simulink model "model"  (R2014a)
(part 5 of 5)

      | %<Vbase>V
      | %<VLF>pu
      | %<angleLF>deg.
      | %<Name>
  bus38 : powerlib/Measurements/Load Flow Bus  LConnTagsString=a  ID=bus38  Vbase=230000  Vref=1  Vangle=0  VLF=1  angleLF=0
      settings: AttributesFormatString=|
      | %<ID>
      | %<Vbase>V
      | %<VLF>pu
      | %<angleLF>deg.
      | %<Name>
  bus39 : powerlib/Measurements/Load Flow Bus  LConnTagsString=a  ID=bus39  Vbase=230000  Vref=1  Vangle=0  VLF=1  angleLF=0
      settings: AttributesFormatString=|
      | %<ID>
      | %<Vbase>V
      | %<VLF>pu
      | %<angleLF>deg.
      | %<Name>
  bus4 : powerlib/Measurements/Load Flow Bus  LConnTagsString=a  ID=bus4  Vbase=66000  Vref=1  Vangle=0  VLF=1  angleLF=0
      settings: AttributesFormatString=|
      | %<ID>
      | %<Vbase>V
      | %<VLF>pu
      | %<angleLF>deg.
      | %<Name>
  bus40 : powerlib/Measurements/Load Flow Bus  LConnTagsString=a  ID=bus40  Vbase=230000  Vref=1  Vangle=0  VLF=1  angleLF=0
      settings: AttributesFormatString=|
      | %<ID>
      | %<Vbase>V
      | %<VLF>pu
      | %<angleLF>deg.
      | %<Name>
  bus41 : powerlib/Measurements/Load Flow Bus  LConnTagsString=a  ID=bus41  Vbase=230000  Vref=1  Vangle=0  VLF=1  angleLF=0
      settings: AttributesFormatString=|
      | %<ID>
      | %<Vbase>V
      | %<VLF>pu
      | %<angleLF>deg.
      | %<Name>
  bus42 : powerlib/Measurements/Load Flow Bus  LConnTagsString=a  ID=bus42  Vbase=230000  Vref=1  Vangle=0  VLF=1  angleLF=0
      settings: AttributesFormatString=|
      | %<ID>
      | %<Vbase>V
      | %<VLF>pu
      | %<angleLF>deg.
      | %<Name>
  bus43 : powerlib/Measurements/Load Flow Bus  LConnTagsString=a  ID=bus43  Vbase=230000  Vref=1  Vangle=0  VLF=1  angleLF=0
      settings: AttributesFormatString=|
      | %<ID>
      | %<Vbase>V
      | %<VLF>pu
      | %<angleLF>deg.
      | %<Name>
  bus44 : powerlib/Measurements/Load Flow Bus  LConnTagsString=a  ID=bus44  Vbase=230000  Vref=1  Vangle=0  VLF=1  angleLF=0
      settings: AttributesFormatString=|
      | %<ID>
      | %<Vbase>V
      | %<VLF>pu
      | %<angleLF>deg.
      | %<Name>
  bus45 : powerlib/Measurements/Load Flow Bus  LConnTagsString=a  ID=bus45  Vbase=230000  Vref=1  Vangle=0  VLF=1  angleLF=0
      settings: AttributesFormatString=|
      | %<ID>
      | %<Vbase>V
      | %<VLF>pu
      | %<angleLF>deg.
      | %<Name>
  bus46 : powerlib/Measurements/Load Flow Bus  LConnTagsString=a  ID=bus46  Vbase=230000  Vref=1  Vangle=0  VLF=1  angleLF=0
      settings: AttributesFormatString=|
      | %<ID>
      | %<Vbase>V
      | %<VLF>pu
      | %<angleLF>deg.
      | %<Name>
  bus47 : powerlib/Measurements/Load Flow Bus  LConnTagsString=a  ID=bus47  Vbase=230000  Vref=1  Vangle=0  VLF=1  angleLF=0
      settings: AttributesFormatString=|
      | %<ID>
      | %<Vbase>V
      | %<VLF>pu
      | %<angleLF>deg.
      | %<Name>
  bus48 : powerlib/Measurements/Load Flow Bus  LConnTagsString=a  ID=bus48  Vbase=230000  Vref=1  Vangle=0  VLF=1  angleLF=0
      settings: AttributesFormatString=|
      | %<ID>
      | %<Vbase>V
      | %<VLF>pu
      | %<angleLF>deg.
      | %<Name>
  bus49 : powerlib/Measurements/Load Flow Bus  LConnTagsString=a  ID=bus49  Vbase=230000  Vref=1  Vangle=0  VLF=1  angleLF=0
      settings: AttributesFormatString=|
      | %<ID>
      | %<Vbase>V
      | %<VLF>pu
      | %<angleLF>deg.
      | %<Name>
  bus5 : powerlib/Measurements/Load Flow Bus  LConnTagsString=a  ID=bus5  Vbase=66000  Vref=1  Vangle=0  VLF=1  angleLF=0
      settings: AttributesFormatString=|
      | %<ID>
      | %<Vbase>V
      | %<VLF>pu
      | %<angleLF>deg.
      | %<Name>
  bus50 : powerlib/Measurements/Load Flow Bus  LConnTagsString=a  ID=bus50  Vbase=230000  Vref=1  Vangle=0  VLF=1  angleLF=0
      settings: AttributesFormatString=|
      | %<ID>
      | %<Vbase>V
      | %<VLF>pu
      | %<angleLF>deg.
      | %<Name>
  bus51 : powerlib/Measurements/Load Flow Bus  LConnTagsString=a  ID=bus51  Vbase=230000  Vref=1  Vangle=0  VLF=1  angleLF=0
      settings: AttributesFormatString=|
      | %<ID>
      | %<Vbase>V
      | %<VLF>pu
      | %<angleLF>deg.
      | %<Name>
  bus52 : powerlib/Measurements/Load Flow Bus  LConnTagsString=a  ID=bus52  Vbase=230000  Vref=1  Vangle=0  VLF=1  angleLF=0
      settings: AttributesFormatString=|
      | %<ID>
      | %<Vbase>V
      | %<VLF>pu
      | %<angleLF>deg.
      | %<Name>
  bus53 : powerlib/Measurements/Load Flow Bus  LConnTagsString=a  ID=bus53  Vbase=230000  Vref=1  Vangle=0  VLF=1  angleLF=0
      settings: AttributesFormatString=|
      | %<ID>
      | %<Vbase>V
      | %<VLF>pu
      | %<angleLF>deg.
      | %<Name>
  bus54 : powerlib/Measurements/Load Flow Bus  LConnTagsString=a  ID=bus54  Vbase=230000  Vref=1  Vangle=0  VLF=1  angleLF=0
      settings: AttributesFormatString=|
      | %<ID>
      | %<Vbase>V
      | %<VLF>pu
      | %<angleLF>deg.
      | %<Name>
  bus55 : powerlib/Measurements/Load Flow Bus  LConnTagsString=a  ID=bus55  Vbase=230000  Vref=1  Vangle=0  VLF=1  angleLF=0
      settings: AttributesFormatString=|
      | %<ID>
      | %<Vbase>V
      | %<VLF>pu
      | %<angleLF>deg.
      | %<Name>
  bus56 : powerlib/Measurements/Load Flow Bus  LConnTagsString=a  ID=bus56  Vbase=230000  Vref=1  Vangle=0  VLF=1  angleLF=0
      settings: AttributesFormatString=|
      | %<ID>
      | %<Vbase>V
      | %<VLF>pu
      | %<angleLF>deg.
      | %<Name>
  bus57 : powerlib/Measurements/Load Flow Bus  LConnTagsString=a  ID=bus57  Vbase=230000  Vref=1  Vangle=0  VLF=1  angleLF=0
      settings: AttributesFormatString=|
      | %<ID>
      | %<Vbase>V
      | %<VLF>pu
      | %<angleLF>deg.
      | %<Name>
  bus58 : powerlib/Measurements/Load Flow Bus  LConnTagsString=a  ID=bus58  Vbase=230000  Vref=1  Vangle=0  VLF=1  angleLF=0
      settings: AttributesFormatString=|
      | %<ID>
      | %<Vbase>V
      | %<VLF>pu
      | %<angleLF>deg.
      | %<Name>
  bus59 : powerlib/Measurements/Load Flow Bus  LConnTagsString=a  ID=bus59  Vbase=230000  Vref=1  Vangle=0  VLF=1  angleLF=0
      settings: AttributesFormatString=|
      | %<ID>
      | %<Vbase>V
      | %<VLF>pu
      | %<angleLF>deg.
      | %<Name>
  bus6 : powerlib/Measurements/Load Flow Bus  LConnTagsString=a  ID=bus6  Vbase=66000  Vref=1  Vangle=0  VLF=1  angleLF=0
      settings: AttributesFormatString=|
      | %<ID>
      | %<Vbase>V
      | %<VLF>pu
      | %<angleLF>deg.
      | %<Name>
  bus60 : powerlib/Measurements/Load Flow Bus  LConnTagsString=a  ID=bus60  Vbase=230000  Vref=1  Vangle=0  VLF=1  angleLF=0
      settings: AttributesFormatString=|
      | %<ID>
      | %<Vbase>V
      | %<VLF>pu
      | %<angleLF>deg.
      | %<Name>
  bus61 : powerlib/Measurements/Load Flow Bus  LConnTagsString=a  ID=bus61  Vbase=230000  Vref=1  Vangle=0  VLF=1  angleLF=0
      settings: AttributesFormatString=|
      | %<ID>
      | %<Vbase>V
      | %<VLF>pu
      | %<angleLF>deg.
      | %<Name>
  bus62 : powerlib/Measurements/Load Flow Bus  LConnTagsString=a  ID=bus62  Vbase=230000  Vref=1  Vangle=0  VLF=1  angleLF=0
      settings: AttributesFormatString=|
      | %<ID>
      | %<Vbase>V
      | %<VLF>pu
      | %<angleLF>deg.
      | %<Name>
  bus63 : powerlib/Measurements/Load Flow Bus  LConnTagsString=a  ID=bus63  Vbase=230000  Vref=1  Vangle=0  VLF=1  angleLF=0
      settings: AttributesFormatString=|
      | %<ID>
      | %<Vbase>V
      | %<VLF>pu
      | %<angleLF>deg.
      | %<Name>
  bus64 : powerlib/Measurements/Load Flow Bus  LConnTagsString=a  ID=bus64  Vbase=230000  Vref=1  Vangle=0  VLF=1  angleLF=0
      settings: AttributesFormatString=|
      | %<ID>
      | %<Vbase>V
      | %<VLF>pu
      | %<angleLF>deg.
      | %<Name>
  bus65 : powerlib/Measurements/Load Flow Bus  LConnTagsString=a  ID=bus65  Vbase=230000  Vref=1  Vangle=0  VLF=1  angleLF=0
      settings: AttributesFormatString=|
      | %<ID>
      | %<Vbase>V
      | %<VLF>pu
      | %<angleLF>deg.
      | %<Name>
  bus66 : powerlib/Measurements/Load Flow Bus  LConnTagsString=a  ID=bus66  Vbase=230000  Vref=1  Vangle=0  VLF=1  angleLF=0
      settings: AttributesFormatString=|
      | %<ID>
      | %<Vbase>V
      | %<VLF>pu
      | %<angleLF>deg.
      | %<Name>
  bus67 : powerlib/Measurements/Load Flow Bus  LConnTagsString=a  ID=bus67  Vbase=230000  Vref=1  Vangle=0  VLF=1  angleLF=0
      settings: AttributesFormatString=|
      | %<ID>
      | %<Vbase>V
      | %<VLF>pu
      | %<angleLF>deg.
      | %<Name>
  bus68 : powerlib/Measurements/Load Flow Bus  LConnTagsString=a  ID=bus68  Vbase=230000  Vref=1  Vangle=0  VLF=1  angleLF=0
      settings: AttributesFormatString=|
      | %<ID>
      | %<Vbase>V
      | %<VLF>pu
      | %<angleLF>deg.
      | %<Name>
  bus69 : powerlib/Measurements/Load Flow Bus  LConnTagsString=a  ID=bus69  Vbase=230000  Vref=1  Vangle=0  VLF=1  angleLF=0
      settings: AttributesFormatString=|
      | %<ID>
      | %<Vbase>V
      | %<VLF>pu
      | %<angleLF>deg.
      | %<Name>
  bus7 : powerlib/Measurements/Load Flow Bus  LConnTagsString=a  ID=bus7  Vbase=66000  Vref=1  Vangle=0  VLF=1  angleLF=0
      settings: AttributesFormatString=|
      | %<ID>
      | %<Vbase>V
      | %<VLF>pu
      | %<angleLF>deg.
      | %<Name>
  bus70 : powerlib/Measurements/Load Flow Bus  LConnTagsString=a  ID=bus70  Vbase=230000  Vref=1  Vangle=0  VLF=1  angleLF=0
      settings: AttributesFormatString=|
      | %<ID>
      | %<Vbase>V
      | %<VLF>pu
      | %<angleLF>deg.
      | %<Name>
  bus71 : powerlib/Measurements/Load Flow Bus  LConnTagsString=a  ID=bus71  Vbase=230000  Vref=1  Vangle=0  VLF=1  angleLF=0
      settings: AttributesFormatString=|
      | %<ID>
      | %<Vbase>V
      | %<VLF>pu
      | %<angleLF>deg.
      | %<Name>
  bus72 : powerlib/Measurements/Load Flow Bus  LConnTagsString=a  ID=bus72  Vbase=230000  Vref=1  Vangle=0  VLF=1  angleLF=0
      settings: AttributesFormatString=|
      | %<ID>
      | %<Vbase>V
      | %<VLF>pu
      | %<angleLF>deg.
      | %<Name>
  bus73 : powerlib/Measurements/Load Flow Bus  LConnTagsString=a  ID=bus73  Vbase=230000  Vref=1  Vangle=0  VLF=1  angleLF=0
      settings: AttributesFormatString=|
      | %<ID>
      | %<Vbase>V
      | %<VLF>pu
      | %<angleLF>deg.
      | %<Name>
  bus74 : powerlib/Measurements/Load Flow Bus  LConnTagsString=a  ID=bus74  Vbase=230000  Vref=1  Vangle=0  VLF=1  angleLF=0
      settings: AttributesFormatString=|
      | %<ID>
      | %<Vbase>V
      | %<VLF>pu
      | %<angleLF>deg.
      | %<Name>
  bus75 : powerlib/Measurements/Load Flow Bus  LConnTagsString=a  ID=bus75  Vbase=230000  Vref=1  Vangle=0  VLF=1  angleLF=0
      settings: AttributesFormatString=|
      | %<ID>
      | %<Vbase>V
      | %<VLF>pu
      | %<angleLF>deg.
      | %<Name>
  bus76 : powerlib/Measurements/Load Flow Bus  LConnTagsString=a  ID=bus76  Vbase=230000  Vref=1  Vangle=0  VLF=1  angleLF=0
      settings: AttributesFormatString=|
      | %<ID>
      | %<Vbase>V
      | %<VLF>pu
      | %<angleLF>deg.
      | %<Name>
  bus77 : powerlib/Measurements/Load Flow Bus  LConnTagsString=a  ID=bus77  Vbase=230000  Vref=1  Vangle=0  VLF=1  angleLF=0
      settings: AttributesFormatString=|
      | %<ID>
      | %<Vbase>V
      | %<VLF>pu
      | %<angleLF>deg.
      | %<Name>
  bus78 : powerlib/Measurements/Load Flow Bus  LConnTagsString=a  ID=bus78  Vbase=230000  Vref=1  Vangle=0  VLF=1  angleLF=0
      settings: AttributesFormatString=|
      | %<ID>
      | %<Vbase>V
      | %<VLF>pu
      | %<angleLF>deg.
      | %<Name>
  bus79 : powerlib/Measurements/Load Flow Bus  LConnTagsString=a  ID=bus79  Vbase=230000  Vref=1  Vangle=0  VLF=1  angleLF=0
      settings: AttributesFormatString=|
      | %<ID>
      | %<Vbase>V
      | %<VLF>pu
      | %<angleLF>deg.
      | %<Name>
  bus8 : powerlib/Measurements/Load Flow Bus  LConnTagsString=a  ID=bus8  Vbase=66000  Vref=1  Vangle=0  VLF=1  angleLF=0
      settings: AttributesFormatString=|
      | %<ID>
      | %<Vbase>V
      | %<VLF>pu
      | %<angleLF>deg.
      | %<Name>
  bus80 : powerlib/Measurements/Load Flow Bus  LConnTagsString=a  ID=bus80  Vbase=230000  Vref=1  Vangle=0  VLF=1  angleLF=0
      settings: AttributesFormatString=|
      | %<ID>
      | %<Vbase>V
      | %<VLF>pu
      | %<angleLF>deg.
      | %<Name>
  bus81 : powerlib/Measurements/Load Flow Bus  LConnTagsString=a  ID=bus81  Vbase=230000  Vref=1  Vangle=0  VLF=1  angleLF=0
      settings: AttributesFormatString=|
      | %<ID>
      | %<Vbase>V
      | %<VLF>pu
      | %<angleLF>deg.
      | %<Name>
  bus82 : powerlib/Measurements/Load Flow Bus  LConnTagsString=a  ID=bus82  Vbase=230000  Vref=1  Vangle=0  VLF=1  angleLF=0
      settings: AttributesFormatString=|
      | %<ID>
      | %<Vbase>V
      | %<VLF>pu
      | %<angleLF>deg.
      | %<Name>
  bus83 : powerlib/Measurements/Load Flow Bus  LConnTagsString=a  ID=bus83  Vbase=230000  Vref=1  Vangle=0  VLF=1  angleLF=0
      settings: AttributesFormatString=|
      | %<ID>
      | %<Vbase>V
      | %<VLF>pu
      | %<angleLF>deg.
      | %<Name>
  bus84 : powerlib/Measurements/Load Flow Bus  LConnTagsString=a  ID=bus84  Vbase=230000  Vref=1  Vangle=0  VLF=1  angleLF=0
      settings: AttributesFormatString=|
      | %<ID>
      | %<Vbase>V
      | %<VLF>pu
      | %<angleLF>deg.
      | %<Name>
  bus85 : powerlib/Measurements/Load Flow Bus  LConnTagsString=a  ID=bus85  Vbase=230000  Vref=1  Vangle=0  VLF=1  angleLF=0
      settings: AttributesFormatString=|
      | %<ID>
      | %<Vbase>V
      | %<VLF>pu
      | %<angleLF>deg.
      | %<Name>
  bus86 : powerlib/Measurements/Load Flow Bus  LConnTagsString=a  ID=bus86  Vbase=400000  Vref=1  Vangle=0  VLF=1  angleLF=0
      settings: AttributesFormatString=|
      | %<ID>
      | %<Vbase>V
      | %<VLF>pu
      | %<angleLF>deg.
      | %<Name>
  bus87 : powerlib/Measurements/Load Flow Bus  LConnTagsString=a  ID=bus87  Vbase=400000  Vref=1  Vangle=0  VLF=1  angleLF=0
      settings: AttributesFormatString=|
      | %<ID>
      | %<Vbase>V
      | %<VLF>pu
      | %<angleLF>deg.
      | %<Name>
  bus88 : powerlib/Measurements/Load Flow Bus  LConnTagsString=a  ID=bus88  Vbase=400000  Vref=1  Vangle=0  VLF=1  angleLF=0
      settings: AttributesFormatString=|
      | %<ID>
      | %<Vbase>V
      | %<VLF>pu
      | %<angleLF>deg.
      | %<Name>
  bus89 : powerlib/Measurements/Load Flow Bus  LConnTagsString=a  ID=bus89  Vbase=400000  Vref=1  Vangle=0  VLF=1  angleLF=0
      settings: AttributesFormatString=|
      | %<ID>
      | %<Vbase>V
      | %<VLF>pu
      | %<angleLF>deg.
      | %<Name>
  bus9 : powerlib/Measurements/Load Flow Bus  LConnTagsString=a  ID=bus9  Vbase=66000  Vref=1  Vangle=0  VLF=1  angleLF=0
      settings: AttributesFormatString=|
      | %<ID>
      | %<Vbase>V
      | %<VLF>pu
      | %<angleLF>deg.
      | %<Name>
  bus90 : powerlib/Measurements/Load Flow Bus  LConnTagsString=a  ID=bus90  Vbase=400000  Vref=1  Vangle=0  VLF=1  angleLF=0
      settings: AttributesFormatString=|
      | %<ID>
      | %<Vbase>V
      | %<VLF>pu
      | %<angleLF>deg.
      | %<Name>
  bus91 : powerlib/Measurements/Load Flow Bus  LConnTagsString=a  ID=bus91  Vbase=400000  Vref=1  Vangle=0  VLF=1  angleLF=0
      settings: AttributesFormatString=|
      | %<ID>
      | %<Vbase>V
      | %<VLF>pu
      | %<angleLF>deg.
      | %<Name>
  bus92 : powerlib/Measurements/Load Flow Bus  LConnTagsString=a  ID=bus92  Vbase=400000  Vref=1  Vangle=0  VLF=1  angleLF=0
      settings: AttributesFormatString=|
      | %<ID>
      | %<Vbase>V
      | %<VLF>pu
      | %<angleLF>deg.
      | %<Name>
  bus93 : powerlib/Measurements/Load Flow Bus  LConnTagsString=a  ID=bus93  Vbase=400000  Vref=1  Vangle=0  VLF=1  angleLF=0
      settings: AttributesFormatString=|
      | %<ID>
      | %<Vbase>V
      | %<VLF>pu
      | %<angleLF>deg.
      | %<Name>
  bus94 : powerlib/Measurements/Load Flow Bus  LConnTagsString=a  ID=bus94  Vbase=400000  Vref=1  Vangle=0  VLF=1  angleLF=0
      settings: AttributesFormatString=|
      | %<ID>
      | %<Vbase>V
      | %<VLF>pu
      | %<angleLF>deg.
      | %<Name>
  bus95 : powerlib/Measurements/Load Flow Bus  LConnTagsString=a  ID=bus95  Vbase=400000  Vref=1  Vangle=0  VLF=1  angleLF=0
      settings: AttributesFormatString=|
      | %<ID>
      | %<Vbase>V
      | %<VLF>pu
      | %<angleLF>deg.
      | %<Name>
  bus96 : powerlib/Measurements/Load Flow Bus  LConnTagsString=a  ID=bus96  Vbase=400000  Vref=1  Vangle=0  VLF=1  angleLF=0
      settings: AttributesFormatString=|
      | %<ID>
      | %<Vbase>V
      | %<VLF>pu
      | %<angleLF>deg.
      | %<Name>
  bus97 : powerlib/Measurements/Load Flow Bus  LConnTagsString=a  ID=bus97  Vbase=400000  Vref=1  Vangle=0  VLF=1  angleLF=0
      settings: AttributesFormatString=|
      | %<ID>
      | %<Vbase>V
      | %<VLF>pu
      | %<angleLF>deg.
      | %<Name>
  bus98 : powerlib/Measurements/Load Flow Bus  LConnTagsString=a  ID=bus98  Vbase=400000  Vref=1  Vangle=0  VLF=1  angleLF=0
      settings: AttributesFormatString=|
      | %<ID>
      | %<Vbase>V
      | %<VLF>pu
      | %<angleLF>deg.
      | %<Name>
  bus99 : powerlib/Measurements/Load Flow Bus  LConnTagsString=a  ID=bus99  Vbase=66000  Vref=1  Vangle=0  VLF=1  angleLF=0
      settings: AttributesFormatString=|
      | %<ID>
      | %<Vbase>V
      | %<VLF>pu
      | %<angleLF>deg.
      | %<Name>
  powergui : powerlib/powergui  Priority=1  SimulationMode=Continuous  SolverType=Tustin  SampleTime=50e-6  frequency=60  SPID=off  DisableSnubberDevices=off  DisableRonSwitches=off  DisableVfSwitches=off  SwTol=0  Interpol=off  DisplayEquations=off  Ts=0  methode=off  frequencyindice=60  Pbase=100e6  ErrMax=1e-4  Iterations=50  UnitsV=kV  UnitsW=MW  FunctionMessages=off  echomessages=off  HookPort=off  EnableUseOfTLC=off  x0status=blocks  RestoreLinks=warning  ResistiveCurrentMeasurement=off  Frange=[0:2:500]  Ylog=off  Xlog=on  ShowGrid=off  save=off  variable=ZData  structure=0  ZoomFFT=off  StartTime=0.0  cycles=1  DisplayStyle=1  fundamental=60  FreqAxis=off  MaxFrequency=1000  frequencyindicesteady=1  RmsSteady=1  display=off
  Ötztal___Zirl_CN_147563007_110000_CN_100404264_110000 : powerlib/Elements/Distributed Parameters Line  Phases=3  Frequency=60  Resistance=[0.01273 0.3864]  Inductance="[0.9337e-3  4.1264e-3]"  Capacitance=[12.74e-9 7.751e-9]  Length=100  x1=[0 0 0 0; 0.0001244 0 0 0; 0.0002488 0 0 0; 0.0003733 0 0 0; 0.0004977 0 0 0; 0.0006221 0 0 0]  x2=[0 0 0 0; 0.0001244 0 0 0; 0.0002488 0 0 0; 0.0003733 0 0 0; 0.0004977 0 0 0; 0.0006221 0 0 0]  x3=[0 0 0 0; 0.0001244 0 0 0; 0.0002488 0 0 0; 0.0003733 0 0 0; 0.0004977 0 0 0; 0.0006221 0 0 0]  x4=[0 0 0 0; 0.0001244 0 0 0; 0.0002488 0 0 0; 0.0003733 0 0 0; 0.0004977 0 0 0; 0.0006221 0 0 0]  x5=0  V1=ones(3,3)  V2=ones(3,3)  I1=ones(3,3)  I2=ones(3,3)  nHarmo=1  Measurements=None
  connections:
  T_172436615__/LConn1 -- _CN_172436615_66000_CN_150358740_66000/LConn1
  T_172436615__/LConn2 -- _CN_172436615_66000_CN_150358740_66000/LConn2
  _CN_172436615_66000_CN_150358740_66000/LConn3 -- T_172436615__/LConn3 -- bus1/LConn1
  _CN_172436615_66000_CN_150358740_66000/RConn1 -- T_150358740__/LConn1 -- _CN_153750231_66000_CN_150358740_66000/LConn1
  _CN_172436615_66000_CN_150358740_66000/RConn2 -- T_150358740__/LConn2 -- _CN_153750231_66000_CN_150358740_66000/LConn2
  _CN_172436615_66000_CN_150358740_66000/RConn3 -- T_150358740__/LConn3 -- _CN_153750231_66000_CN_150358740_66000/LConn3 -- bus2/LConn1
  _CN_152303368_66000_CN_152303372_66000/LConn1 -- T_152303368__/LConn1 -- _CN_152303368_66000_CN_152322299_66000/LConn1
  _CN_152303368_66000_CN_152303372_66000/LConn2 -- T_152303368__/LConn2 -- _CN_152303368_66000_CN_152322299_66000/LConn2
  _CN_152303368_66000_CN_152303372_66000/LConn3 -- T_152303368__/LConn3 -- _CN_152303368_66000_CN_152322299_66000/LConn3 -- bus3/LConn1
  _CN_152303368_66000_CN_152303372_66000/RConn1 -- T_152303372__/RConn1 -- _CN_152303372_66000_CN_154474061_66000/LConn1 -- _CN_152303372_66000_CN_150256289_66000/LConn1 -- L_152303372/LConn1
  _CN_152303368_66000_CN_152303372_66000/RConn2 -- T_152303372__/RConn2 -- _CN_152303372_66000_CN_154474061_66000/LConn2 -- _CN_152303372_66000_CN_150256289_66000/LConn2 -- L_152303372/LConn2
  _CN_152303368_66000_CN_152303372_66000/RConn3 -- T_152303372__/RConn3 -- _CN_152303372_66000_CN_154474061_66000/LConn3 -- _CN_152303372_66000_CN_150256289_66000/LConn3 -- L_152303372/LConn3 -- bus4/LConn1
  T_152322299__/LConn1 -- _CN_152303368_66000_CN_152322299_66000/RConn1
  T_152322299__/LConn2 -- _CN_152303368_66000_CN_152322299_66000/RConn2
  _CN_152303368_66000_CN_152322299_66000/RConn3 -- T_152322299__/LConn3 -- bus5/LConn1
  _CN_130804490_66000_CN_223610661_66000/LConn1 -- T_130804490__/RConn1 -- _CN_130804490_66000_CN_130790482_66000/LConn1 -- _CN_130804490_66000_CN_382319714_66000/LConn1 -- L_130804490/LConn1
  _CN_130804490_66000_CN_223610661_66000/LConn2 -- T_130804490__/RConn2 -- _CN_130804490_66000_CN_130790482_66000/LConn2 -- _CN_130804490_66000_CN_382319714_66000/LConn2 -- L_130804490/LConn2
  _CN_130804490_66000_CN_223610661_66000/LConn3 -- T_130804490__/RConn3 -- _CN_130804490_66000_CN_130790482_66000/LConn3 -- _CN_130804490_66000_CN_382319714_66000/LConn3 -- L_130804490/LConn3 -- bus6/LConn1
  _CN_130804490_66000_CN_223610661_66000/RConn1 -- T_223610661__/LConn1 -- _CN_130790482_66000_CN_223610661_66000/LConn1
  _CN_130804490_66000_CN_223610661_66000/RConn2 -- T_223610661__/LConn2 -- _CN_130790482_66000_CN_223610661_66000/LConn2
  _CN_130804490_66000_CN_223610661_66000/RConn3 -- T_223610661__/LConn3 -- _CN_130790482_66000_CN_223610661_66000/LConn3 -- bus7/LConn1
  _CN_130804490_66000_CN_130790482_66000/RConn1 -- T_130790482__/LConn1 -- _CN_382484415_66000_CN_130790482_66000/LConn1 -- _CN_130790482_66000_CN_223610661_66000/RConn1 -- _CN_130790482_66000_CN_130805766_66000/LConn1
  _CN_130804490_66000_CN_130790482_66000/RConn2 -- T_130790482__/LConn2 -- _CN_382484415_66000_CN_130790482_66000/LConn2 -- _CN_130790482_66000_CN_223610661_66000/RConn2 -- _CN_130790482_66000_CN_130805766_66000/LConn2
  _CN_130804490_66000_CN_130790482_66000/RConn3 -- T_130790482__/LConn3 -- _CN_382484415_66000_CN_130790482_66000/LConn3 -- _CN_130790482_66000_CN_223610661_66000/RConn3 -- _CN_130790482_66000_CN_130805766_66000/LConn3 -- bus8/LConn1
  T_382319714__/LConn1 -- _CN_130804490_66000_CN_382319714_66000/RConn1
  T_382319714__/LConn2 -- _CN_130804490_66000_CN_382319714_66000/RConn2
  _CN_130804490_66000_CN_382319714_66000/RConn3 -- T_382319714__/LConn3 -- bus9/LConn1
  _CN_130804491_66000_CN_382489138_66000/LConn1 -- T_130804491__/RConn1 -- L_130804491/LConn1
  _CN_130804491_66000_CN_382489138_66000/LConn2 -- T_130804491__/RConn2 -- L_130804491/LConn2
  _CN_130804491_66000_CN_382489138_66000/LConn3 -- T_130804491__/RConn3 -- L_130804491/LConn3 -- bus10/LConn1
  G_382489138_/RConn1 -- _CN_130804491_66000_CN_382489138_66000/RConn1
  G_382489138_/RConn2 -- _CN_130804491_66000_CN_382489138_66000/RConn2
  _CN_130804491_66000_CN_382489138_66000/RConn3 -- G_382489138_/RConn3 -- bus11/LConn1
  T_154474061__/LConn1 -- _CN_152303372_66000_CN_154474061_66000/RConn1
  T_154474061__/LConn2 -- _CN_152303372_66000_CN_154474061_66000/RConn2
  _CN_152303372_66000_CN_154474061_66000/RConn3 -- T_154474061__/LConn3 -- bus12/LConn1
  _CN_152303372_66000_CN_150256289_66000/RConn1 -- T_150256289__/RConn1 -- _CN_150256289_66000_CN_171978321_66000/LConn1 -- L_150256289/LConn1 -- _CN_153750231_66000_CN_150256289_66000/LConn1
  _CN_152303372_66000_CN_150256289_66000/RConn2 -- T_150256289__/RConn2 -- _CN_150256289_66000_CN_171978321_66000/LConn2 -- L_150256289/LConn2 -- _CN_153750231_66000_CN_150256289_66000/LConn2
  _CN_152303372_66000_CN_150256289_66000/RConn3 -- T_150256289__/RConn3 -- _CN_150256289_66000_CN_171978321_66000/LConn3 -- L_150256289/LConn3 -- bus13/LConn1 -- _CN_153750231_66000_CN_150256289_66000/LConn3
  _CN_153750231_66000_CN_150256289_66000/RConn1 -- T_153750231__/LConn1 -- _CN_153750231_66000_CN_150358740_66000/RConn1
  _CN_153750231_66000_CN_150256289_66000/RConn2 -- T_153750231__/LConn2 -- _CN_153750231_66000_CN_150358740_66000/RConn2
  _CN_153750231_66000_CN_150256289_66000/RConn3 -- T_153750231__/LConn3 -- _CN_153750231_66000_CN_150358740_66000/RConn3 -- bus14/LConn1
  T_204550424__/LConn1 -- _CN_204550424_66000_CN_130805766_66000/LConn1
  T_204550424__/LConn2 -- _CN_204550424_66000_CN_130805766_66000/LConn2
  _CN_204550424_66000_CN_130805766_66000/LConn3 -- T_204550424__/LConn3 -- bus15/LConn1
  _CN_204550424_66000_CN_130805766_66000/RConn1 -- G_130805766_/RConn1 -- _CN_130790482_66000_CN_130805766_66000/RConn1 -- _CN_130805767_230000_CN_130805766_66000/LConn1 -- _CN_130804490_230000_CN_130805766_66000/LConn1 -- _CN_130804491_230000_CN_130805766_66000/LConn1 -- _CN_223610662_66000_CN_130805766_66000/LConn1
  _CN_204550424_66000_CN_130805766_66000/RConn2 -- G_130805766_/RConn2 -- _CN_130790482_66000_CN_130805766_66000/RConn2 -- _CN_130805767_230000_CN_130805766_66000/LConn2 -- _CN_130804490_230000_CN_130805766_66000/LConn2 -- _CN_130804491_230000_CN_130805766_66000/LConn2 -- _CN_223610662_66000_CN_130805766_66000/LConn2
  _CN_204550424_66000_CN_130805766_66000/RConn3 -- G_130805766_/RConn3 -- _CN_130790482_66000_CN_130805766_66000/RConn3 -- _CN_130805767_230000_CN_130805766_66000/LConn3 -- _CN_130804490_230000_CN_130805766_66000/LConn3 -- _CN_130804491_230000_CN_130805766_66000/LConn3 -- bus16/LConn1 -- _CN_223610662_66000_CN_130805766_66000/LConn3
  _CN_180326303_66000_CN_180330721_66000/LConn1 -- T_180326303__/RConn1 -- _CN_180326303_66000_CN_368593331_66000/LConn1 -- L_180326303/LConn1
  _CN_180326303_66000_CN_180330721_66000/LConn2 -- T_180326303__/RConn2 -- _CN_180326303_66000_CN_368593331_66000/LConn2 -- L_180326303/LConn2
  _CN_180326303_66000_CN_180330721_66000/LConn3 -- T_180326303__/RConn3 -- _CN_180326303_66000_CN_368593331_66000/LConn3 -- L_180326303/LConn3 -- bus17/LConn1
  T_180330721__/LConn1 -- _CN_180326303_66000_CN_180330721_66000/RConn1
  T_180330721__/LConn2 -- _CN_180326303_66000_CN_180330721_66000/RConn2
  _CN_180326303_66000_CN_180330721_66000/RConn3 -- T_180330721__/LConn3 -- bus18/LConn1
  T_368593331__/LConn1 -- _CN_180326303_66000_CN_368593331_66000/RConn1
  T_368593331__/LConn2 -- _CN_180326303_66000_CN_368593331_66000/RConn2
  _CN_180326303_66000_CN_368593331_66000/RConn3 -- T_368593331__/LConn3 -- bus19/LConn1
  _CN_150256289_66000_CN_171978321_66000/RConn1 -- T_171978321__/LConn1 -- _CN_171978319_66000_CN_171978321_66000/LConn1
  _CN_150256289_66000_CN_171978321_66000/RConn2 -- T_171978321__/LConn2 -- _CN_171978319_66000_CN_171978321_66000/LConn2
  _CN_150256289_66000_CN_171978321_66000/RConn3 -- T_171978321__/LConn3 -- _CN_171978319_66000_CN_171978321_66000/LConn3 -- bus20/LConn1
  _CN_167991716_66000_CN_157393020_66000/LConn1 -- T_167991716_66000_/LConn1 -- _CN_167991716_66000_CN_157858216_66000/LConn1
  _CN_167991716_66000_CN_157393020_66000/LConn2 -- T_167991716_66000_/LConn2 -- _CN_167991716_66000_CN_157858216_66000/LConn2
  _CN_167991716_66000_CN_157393020_66000/LConn3 -- T_167991716_66000_/LConn3 -- _CN_167991716_66000_CN_157858216_66000/LConn3 -- bus21/LConn1
  T_157393020__/LConn1 -- _CN_167991716_66000_CN_157393020_66000/RConn1
  T_157393020__/LConn2 -- _CN_167991716_66000_CN_157393020_66000/RConn2
  _CN_167991716_66000_CN_157393020_66000/RConn3 -- T_157393020__/LConn3 -- bus22/LConn1
  _CN_167991716_66000_CN_157858216_66000/RConn1 -- T_157858216_230000;66000_/RConn1 -- L_157858216/LConn1
  _CN_167991716_66000_CN_157858216_66000/RConn2 -- T_157858216_230000;66000_/RConn2 -- L_157858216/LConn2
  _CN_167991716_66000_CN_157858216_66000/RConn3 -- T_157858216_230000;66000_/RConn3 -- L_157858216/LConn3 -- bus23/LConn1
  _CN_223610662_66000_CN_130805766_66000/RConn1 -- T_223610662__/LConn1 -- _CN_223610662_66000_CN_382300120_66000/LConn1
  _CN_223610662_66000_CN_130805766_66000/RConn2 -- T_223610662__/LConn2 -- _CN_223610662_66000_CN_382300120_66000/LConn2
  _CN_223610662_66000_CN_130805766_66000/RConn3 -- T_223610662__/LConn3 -- _CN_223610662_66000_CN_382300120_66000/LConn3 -- bus24/LConn1
  T_382300120__/LConn1 -- _CN_223610662_66000_CN_382300120_66000/RConn1
  T_382300120__/LConn2 -- _CN_223610662_66000_CN_382300120_66000/RConn2
  _CN_223610662_66000_CN_382300120_66000/RConn3 -- T_382300120__/LConn3 -- bus25/LConn1
  T_382331561__/LConn1 -- _CN_382331561_66000_CN_131421941_66000/LConn1
  T_382331561__/LConn2 -- _CN_382331561_66000_CN_131421941_66000/LConn2
  _CN_382331561_66000_CN_131421941_66000/LConn3 -- T_382331561__/LConn3 -- bus26/LConn1
  _CN_382331561_66000_CN_131421941_66000/RConn1 -- T_131421941__/RConn1 -- L_131421941/LConn1
  _CN_382331561_66000_CN_131421941_66000/RConn2 -- T_131421941__/RConn2 -- L_131421941/LConn2
  _CN_382331561_66000_CN_131421941_66000/RConn3 -- T_131421941__/RConn3 -- L_131421941/LConn3 -- bus27/LConn1
  _CN_238298034_66000_CN_382898922_66000/LConn1 -- T_238298034__/RConn1 -- L_238298034/LConn1
  _CN_238298034_66000_CN_382898922_66000/LConn2 -- T_238298034__/RConn2 -- L_238298034/LConn2
  _CN_238298034_66000_CN_382898922_66000/LConn3 -- T_238298034__/RConn3 -- L_238298034/LConn3 -- bus28/LConn1
  T_382898922__/LConn1 -- _CN_238298034_66000_CN_382898922_66000/RConn1
  T_382898922__/LConn2 -- _CN_238298034_66000_CN_382898922_66000/RConn2
  _CN_238298034_66000_CN_382898922_66000/RConn3 -- T_382898922__/LConn3 -- bus29/LConn1
  T_382484415__/LConn1 -- _CN_382484415_66000_CN_130790482_66000/RConn1
  T_382484415__/LConn2 -- _CN_382484415_66000_CN_130790482_66000/RConn2
  _CN_382484415_66000_CN_130790482_66000/RConn3 -- T_382484415__/LConn3 -- bus30/LConn1
  _CN_150974532_66000_CN_155496431_66000/LConn1 -- T_150974532__/RConn1 -- L_150974532/LConn1
  _CN_150974532_66000_CN_155496431_66000/LConn2 -- T_150974532__/RConn2 -- L_150974532/LConn2
  _CN_150974532_66000_CN_155496431_66000/LConn3 -- T_150974532__/RConn3 -- L_150974532/LConn3 -- bus31/LConn1
  T_155496431__/LConn1 -- _CN_150974532_66000_CN_155496431_66000/RConn1
  T_155496431__/LConn2 -- _CN_150974532_66000_CN_155496431_66000/RConn2
  _CN_150974532_66000_CN_155496431_66000/RConn3 -- T_155496431__/LConn3 -- bus32/LConn1
  T_171978319__/LConn1 -- _CN_171978319_66000_CN_171978321_66000/RConn1
  T_171978319__/LConn2 -- _CN_171978319_66000_CN_171978321_66000/RConn2
  _CN_171978319_66000_CN_171978321_66000/RConn3 -- T_171978319__/LConn3 -- bus33/LConn1
  _CN_133331795_66000_CN_160840191_66000/LConn1 -- T_133331795__/RConn1 -- L_133331795/LConn1
  _CN_133331795_66000_CN_160840191_66000/LConn2 -- T_133331795__/RConn2 -- L_133331795/LConn2
  _CN_133331795_66000_CN_160840191_66000/LConn3 -- T_133331795__/RConn3 -- L_133331795/LConn3 -- bus34/LConn1
  T_160840191__/LConn1 -- _CN_133331795_66000_CN_160840191_66000/RConn1
  T_160840191__/LConn2 -- _CN_133331795_66000_CN_160840191_66000/RConn2
  _CN_133331795_66000_CN_160840191_66000/RConn3 -- T_160840191__/LConn3 -- bus35/LConn1
  T_163711729__/LConn1 -- _CN_163711729_66000_CN_110461432_66000/LConn1
  T_163711729__/LConn2 -- _CN_163711729_66000_CN_110461432_66000/LConn2
  _CN_163711729_66000_CN_110461432_66000/LConn3 -- T_163711729__/LConn3 -- bus36/LConn1
  T_110461432__محطة_الكهرباء/LConn1 -- _CN_163711729_66000_CN_110461432_66000/RConn1
  T_110461432__محطة_الكهرباء/LConn2 -- _CN_163711729_66000_CN_110461432_66000/RConn2
  _CN_163711729_66000_CN_110461432_66000/RConn3 -- T_110461432__محطة_الكهرباء/LConn3 -- bus37/LConn1
  _CN_152322304_230000_CN_161969636_230000/LConn1 -- T_152322304__/RConn1 -- L_152322304/LConn1
  _CN_152322304_230000_CN_161969636_230000/LConn2 -- T_152322304__/RConn2 -- L_152322304/LConn2
  _CN_152322304_230000_CN_161969636_230000/LConn3 -- T_152322304__/RConn3 -- L_152322304/LConn3 -- bus38/LConn1
  T_161969636__/LConn1 -- _CN_152322304_230000_CN_161969636_230000/RConn1
  T_161969636__/LConn2 -- _CN_152322304_230000_CN_161969636_230000/RConn2
  _CN_152322304_230000_CN_161969636_230000/RConn3 -- T_161969636__/LConn3 -- bus39/LConn1
  T_164725547__/LConn1 -- _CN_164725547_230000_CN_195237417_230000/LConn1
  T_164725547__/LConn2 -- _CN_164725547_230000_CN_195237417_230000/LConn2
  _CN_164725547_230000_CN_195237417_230000/LConn3 -- T_164725547__/LConn3 -- bus40/LConn1
  T_195237417__/LConn1 -- _CN_164725547_230000_CN_195237417_230000/RConn1
  T_195237417__/LConn2 -- _CN_164725547_230000_CN_195237417_230000/RConn2
  _CN_164725547_230000_CN_195237417_230000/RConn3 -- T_195237417__/LConn3 -- bus41/LConn1
  _CN_130805767_230000_CN_130805766_66000/RConn1 -- T_130805767__/RConn1 -- L_130805767/LConn1
  _CN_130805767_230000_CN_130805766_66000/RConn2 -- T_130805767__/RConn2 -- L_130805767/LConn2
  _CN_130805767_230000_CN_130805766_66000/RConn3 -- T_130805767__/RConn3 -- L_130805767/LConn3 -- bus42/LConn1
  T_152303369__/LConn1 -- _CN_152303369_230000_CN_150638744_230000/LConn1
  T_152303369__/LConn2 -- _CN_152303369_230000_CN_150638744_230000/LConn2
  _CN_152303369_230000_CN_150638744_230000/LConn3 -- T_152303369__/LConn3 -- bus43/LConn1
  _CN_152303369_230000_CN_150638744_230000/RConn1 -- T_150638744__/RConn1 -- _CN_152303372_230000_CN_150638744_230000/LConn1 -- _CN_150638744_230000_CN_150256289_230000/LConn1 -- _CN_150638744_230000_CN_151913391_230000/LConn1 -- _CN_150638744_230000_CN_150358741_230000/LConn1 -- L_150638744/LConn1
  _CN_152303369_230000_CN_150638744_230000/RConn2 -- T_150638744__/RConn2 -- _CN_152303372_230000_CN_150638744_230000/LConn2 -- _CN_150638744_230000_CN_150256289_230000/LConn2 -- _CN_150638744_230000_CN_151913391_230000/LConn2 -- _CN_150638744_230000_CN_150358741_230000/LConn2 -- L_150638744/LConn2
  _CN_152303369_230000_CN_150638744_230000/RConn3 -- T_150638744__/RConn3 -- _CN_152303372_230000_CN_150638744_230000/LConn3 -- _CN_150638744_230000_CN_150256289_230000/LConn3 -- _CN_150638744_230000_CN_151913391_230000/LConn3 -- _CN_150638744_230000_CN_150358741_230000/LConn3 -- L_150638744/LConn3 -- bus44/LConn1
  _CN_130804490_230000_CN_130805766_66000/RConn1 -- T_130804490__/LConn1 -- _CN_130804490_230000_CN_131421941_230000/LConn1
  _CN_130804490_230000_CN_130805766_66000/RConn2 -- T_130804490__/LConn2 -- _CN_130804490_230000_CN_131421941_230000/LConn2
  _CN_130804490_230000_CN_130805766_66000/RConn3 -- T_130804490__/LConn3 -- _CN_130804490_230000_CN_131421941_230000/LConn3 -- bus45/LConn1
  T_131421941__/LConn1 -- _CN_130804490_230000_CN_131421941_230000/RConn1
  T_131421941__/LConn2 -- _CN_130804490_230000_CN_131421941_230000/RConn2
  _CN_130804490_230000_CN_131421941_230000/RConn3 -- T_131421941__/LConn3 -- bus46/LConn1
  _CN_130804491_230000_CN_180326303_230000/LConn1 -- T_130804491__/LConn1 -- _CN_130804491_230000_CN_130805766_66000/RConn1
  _CN_130804491_230000_CN_180326303_230000/LConn2 -- T_130804491__/LConn2 -- _CN_130804491_230000_CN_130805766_66000/RConn2
  _CN_130804491_230000_CN_180326303_230000/LConn3 -- T_130804491__/LConn3 -- _CN_130804491_230000_CN_130805766_66000/RConn3 -- bus47/LConn1
  _CN_130804491_230000_CN_180326303_230000/RConn1 -- T_180326303__/LConn1 -- _CN_180326303_230000_CN_330757612_230000/LConn1 -- _CN_180326303_230000_CN_180326309_230000/LConn1 -- _CN_180326303_230000_CN_113711692_230000/LConn1
  _CN_130804491_230000_CN_180326303_230000/RConn2 -- T_180326303__/LConn2 -- _CN_180326303_230000_CN_330757612_230000/LConn2 -- _CN_180326303_230000_CN_180326309_230000/LConn2 -- _CN_180326303_230000_CN_113711692_230000/LConn2
  _CN_130804491_230000_CN_180326303_230000/RConn3 -- T_180326303__/LConn3 -- _CN_180326303_230000_CN_330757612_230000/LConn3 -- _CN_180326303_230000_CN_180326309_230000/LConn3 -- _CN_180326303_230000_CN_113711692_230000/LConn3 -- bus48/LConn1
  T_152303372__/LConn1 -- _CN_152303372_230000_CN_150638744_230000/RConn1
  T_152303372__/LConn2 -- _CN_152303372_230000_CN_150638744_230000/RConn2
  _CN_152303372_230000_CN_150638744_230000/RConn3 -- T_152303372__/LConn3 -- bus49/LConn1
  _CN_254292628_230000_CN_133424212_230000/LConn1 -- T_254292628__/LConn1 -- _CN_254292628_230000_CN_254292629_230000/LConn1
  _CN_254292628_230000_CN_133424212_230000/LConn2 -- T_254292628__/LConn2 -- _CN_254292628_230000_CN_254292629_230000/LConn2
  _CN_254292628_230000_CN_133424212_230000/LConn3 -- T_254292628__/LConn3 -- _CN_254292628_230000_CN_254292629_230000/LConn3 -- bus50/LConn1
  _CN_254292628_230000_CN_133424212_230000/RConn1 -- T_133424212__/LConn1 -- _CN_133424203_230000_CN_133424212_230000/LConn1 -- _CN_133424212_230000_CN_168164591_230000/LConn1
  _CN_254292628_230000_CN_133424212_230000/RConn2 -- T_133424212__/LConn2 -- _CN_133424203_230000_CN_133424212_230000/LConn2 -- _CN_133424212_230000_CN_168164591_230000/LConn2
  _CN_254292628_230000_CN_133424212_230000/RConn3 -- T_133424212__/LConn3 -- _CN_133424203_230000_CN_133424212_230000/LConn3 -- _CN_133424212_230000_CN_168164591_230000/LConn3 -- bus51/LConn1
  T_254292629__/LConn1 -- _CN_254292628_230000_CN_254292629_230000/RConn1
  T_254292629__/LConn2 -- _CN_254292628_230000_CN_254292629_230000/RConn2
  _CN_254292628_230000_CN_254292629_230000/RConn3 -- T_254292629__/LConn3 -- bus52/LConn1
  _CN_150638744_230000_CN_150256289_230000/RConn1 -- T_150256289__/LConn1 -- _CN_150256289_230000_CN_130593618_230000/LConn1 -- _CN_150256289_230000_CN_150358741_230000/LConn1
  _CN_150638744_230000_CN_150256289_230000/RConn2 -- T_150256289__/LConn2 -- _CN_150256289_230000_CN_130593618_230000/LConn2 -- _CN_150256289_230000_CN_150358741_230000/LConn2
  _CN_150638744_230000_CN_150256289_230000/RConn3 -- T_150256289__/LConn3 -- _CN_150256289_230000_CN_130593618_230000/LConn3 -- _CN_150256289_230000_CN_150358741_230000/LConn3 -- bus53/LConn1
  _CN_150638744_230000_CN_151913391_230000/RConn1 -- T_151913391__/LConn1 -- _CN_151913391_230000_CN_160110669_230000/LConn1
  _CN_150638744_230000_CN_151913391_230000/RConn2 -- T_151913391__/LConn2 -- _CN_151913391_230000_CN_160110669_230000/LConn2
  _CN_150638744_230000_CN_151913391_230000/RConn3 -- T_151913391__/LConn3 -- _CN_151913391_230000_CN_160110669_230000/LConn3 -- bus54/LConn1
  _CN_150638744_230000_CN_150358741_230000/RConn1 -- T_150358741__/LConn1 -- _CN_150256289_230000_CN_150358741_230000/RConn1 -- _CN_150358741_230000_CN_154838308_230000/LConn1 -- _CN_150358741_230000_CN_150579316_230000/LConn1
  _CN_150638744_230000_CN_150358741_230000/RConn2 -- T_150358741__/LConn2 -- _CN_150256289_230000_CN_150358741_230000/RConn2 -- _CN_150358741_230000_CN_154838308_230000/LConn2 -- _CN_150358741_230000_CN_150579316_230000/LConn2
  _CN_150638744_230000_CN_150358741_230000/RConn3 -- T_150358741__/LConn3 -- _CN_150256289_230000_CN_150358741_230000/RConn3 -- _CN_150358741_230000_CN_154838308_230000/LConn3 -- _CN_150358741_230000_CN_150579316_230000/LConn3 -- bus55/LConn1
  _CN_180326303_230000_CN_330757612_230000/RConn1 -- T_330757612__/LConn1 -- _CN_238298034_230000_CN_330757612_230000/LConn1
  _CN_180326303_230000_CN_330757612_230000/RConn2 -- T_330757612__/LConn2 -- _CN_238298034_230000_CN_330757612_230000/LConn2
  _CN_180326303_230000_CN_330757612_230000/RConn3 -- T_330757612__/LConn3 -- _CN_238298034_230000_CN_330757612_230000/LConn3 -- bus56/LConn1
  T_180326309__Electrical_substation/LConn1 -- _CN_180326303_230000_CN_180326309_230000/RConn1
  T_180326309__Electrical_substation/LConn2 -- _CN_180326303_230000_CN_180326309_230000/RConn2
  _CN_180326303_230000_CN_180326309_230000/RConn3 -- T_180326309__Electrical_substation/LConn3 -- bus57/LConn1
  _CN_180326303_230000_CN_113711692_230000/RConn1 -- T_113711692__/LConn1 -- _CN_238298034_230000_CN_113711692_230000/LConn1
  _CN_180326303_230000_CN_113711692_230000/RConn2 -- T_113711692__/LConn2 -- _CN_238298034_230000_CN_113711692_230000/LConn2
  _CN_180326303_230000_CN_113711692_230000/RConn3 -- T_113711692__/LConn3 -- _CN_238298034_230000_CN_113711692_230000/LConn3 -- bus58/LConn1
  _CN_150256289_230000_CN_130593618_230000/RConn1 -- G_130593618_/RConn1 -- _CN_168164591_230000_CN_130593618_230000/LConn1 -- _CN_150974530_400000_CN_130593618_230000/LConn1 -- _CN_150638744_400000_CN_130593618_230000/LConn1 -- _CN_123913890_230000_CN_130593618_230000/LConn1 -- _CN_130592294_230000_CN_130593618_230000/LConn1 -- _CN_124803179_230000_CN_130593618_230000/LConn1
  _CN_150256289_230000_CN_130593618_230000/RConn2 -- G_130593618_/RConn2 -- _CN_168164591_230000_CN_130593618_230000/LConn2 -- _CN_150974530_400000_CN_130593618_230000/LConn2 -- _CN_150638744_400000_CN_130593618_230000/LConn2 -- _CN_123913890_230000_CN_130593618_230000/LConn2 -- _CN_130592294_230000_CN_130593618_230000/LConn2 -- _CN_124803179_230000_CN_130593618_230000/LConn2
  _CN_150256289_230000_CN_130593618_230000/RConn3 -- G_130593618_/RConn3 -- _CN_168164591_230000_CN_130593618_230000/LConn3 -- _CN_150974530_400000_CN_130593618_230000/LConn3 -- _CN_150638744_400000_CN_130593618_230000/LConn3 -- bus59/LConn1 -- _CN_123913890_230000_CN_130593618_230000/LConn3 -- _CN_130592294_230000_CN_130593618_230000/LConn3 -- _CN_124803179_230000_CN_130593618_230000/LConn3
  _CN_123913890_230000_CN_130592294_230000/LConn1 -- T_123913890__/LConn1 -- _CN_123913890_230000_CN_130593618_230000/RConn1
  _CN_123913890_230000_CN_130592294_230000/LConn2 -- T_123913890__/LConn2 -- _CN_123913890_230000_CN_130593618_230000/RConn2
  _CN_123913890_230000_CN_130592294_230000/LConn3 -- T_123913890__/LConn3 -- _CN_123913890_230000_CN_130593618_230000/RConn3 -- bus60/LConn1
  _CN_123913890_230000_CN_130592294_230000/RConn1 -- T_130592294__/LConn1 -- _CN_130592294_230000_CN_133331793_230000/LConn1 -- _CN_130592294_230000_CN_160279731_230000/LConn1 -- _CN_130592294_230000_CN_154838308_230000/LConn1 -- _CN_130592294_230000_CN_130593618_230000/RConn1
  _CN_123913890_230000_CN_130592294_230000/RConn2 -- T_130592294__/LConn2 -- _CN_130592294_230000_CN_133331793_230000/LConn2 -- _CN_130592294_230000_CN_160279731_230000/LConn2 -- _CN_130592294_230000_CN_154838308_230000/LConn2 -- _CN_130592294_230000_CN_130593618_230000/RConn2
  _CN_123913890_230000_CN_130592294_230000/RConn3 -- T_130592294__/LConn3 -- _CN_130592294_230000_CN_133331793_230000/LConn3 -- _CN_130592294_230000_CN_160279731_230000/LConn3 -- _CN_130592294_230000_CN_154838308_230000/LConn3 -- _CN_130592294_230000_CN_130593618_230000/RConn3 -- bus61/LConn1
  _CN_130592294_230000_CN_133331793_230000/RConn1 -- G_133331793_المحطة_الحرارية_Thermal_power_plant/RConn1 -- _CN_133432875_230000_CN_133331793_230000/LConn1 -- _CN_162588721_230000_CN_133331793_230000/LConn1 -- _CN_133331795_230000_CN_133331793_230000/LConn1
  _CN_130592294_230000_CN_133331793_230000/RConn2 -- G_133331793_المحطة_الحرارية_Thermal_power_plant/RConn2 -- _CN_133432875_230000_CN_133331793_230000/LConn2 -- _CN_162588721_230000_CN_133331793_230000/LConn2 -- _CN_133331795_230000_CN_133331793_230000/LConn2
  _CN_130592294_230000_CN_133331793_230000/RConn3 -- G_133331793_المحطة_الحرارية_Thermal_power_plant/RConn3 -- _CN_133432875_230000_CN_133331793_230000/LConn3 -- _CN_162588721_230000_CN_133331793_230000/LConn3 -- _CN_133331795_230000_CN_133331793_230000/LConn3 -- bus62/LConn1
  _CN_130592294_230000_CN_160279731_230000/RConn1 -- T_160279731__/RConn1 -- L_160279731/LConn1
  _CN_130592294_230000_CN_160279731_230000/RConn2 -- T_160279731__/RConn2 -- L_160279731/LConn2
  _CN_130592294_230000_CN_160279731_230000/RConn3 -- T_160279731__/RConn3 -- L_160279731/LConn3 -- bus63/LConn1
  _CN_130592294_230000_CN_154838308_230000/RConn1 -- G_154838308_Al_Zara_Thermal_Power_Plant/RConn1 -- _CN_150358741_230000_CN_154838308_230000/RConn1 -- _CN_124803179_230000_CN_154838308_230000/LConn1
  _CN_130592294_230000_CN_154838308_230000/RConn2 -- G_154838308_Al_Zara_Thermal_Power_Plant/RConn2 -- _CN_150358741_230000_CN_154838308_230000/RConn2 -- _CN_124803179_230000_CN_154838308_230000/LConn2
  _CN_130592294_230000_CN_154838308_230000/RConn3 -- G_154838308_Al_Zara_Thermal_Power_Plant/RConn3 -- _CN_150358741_230000_CN_154838308_230000/RConn3 -- _CN_124803179_230000_CN_154838308_230000/LConn3 -- bus64/LConn1
  _CN_157858216_230000_CN_117335600_230000/LConn1 -- T_157858216_230000;66000_/LConn1 -- _CN_157858216_230000_CN_164701658_230000/LConn1
  _CN_157858216_230000_CN_117335600_230000/LConn2 -- T_157858216_230000;66000_/LConn2 -- _CN_157858216_230000_CN_164701658_230000/LConn2
  _CN_157858216_230000_CN_117335600_230000/LConn3 -- T_157858216_230000;66000_/LConn3 -- _CN_157858216_230000_CN_164701658_230000/LConn3 -- bus65/LConn1
  _CN_157858216_230000_CN_117335600_230000/RConn1 -- T_117335600_400000;230000_/RConn1 -- L_117335600/LConn1
  _CN_157858216_230000_CN_117335600_230000/RConn2 -- T_117335600_400000;230000_/RConn2 -- L_117335600/LConn2
  _CN_157858216_230000_CN_117335600_230000/RConn3 -- T_117335600_400000;230000_/RConn3 -- L_117335600/LConn3 -- bus66/LConn1
  T_164701658__/LConn1 -- _CN_157858216_230000_CN_164701658_230000/RConn1
  T_164701658__/LConn2 -- _CN_157858216_230000_CN_164701658_230000/RConn2
  _CN_157858216_230000_CN_164701658_230000/RConn3 -- T_164701658__/LConn3 -- bus67/LConn1
  T_133432875__/LConn1 -- _CN_133432875_230000_CN_133331793_230000/RConn1
  T_133432875__/LConn2 -- _CN_133432875_230000_CN_133331793_230000/RConn2
  _CN_133432875_230000_CN_133331793_230000/RConn3 -- T_133432875__/LConn3 -- bus68/LConn1
  _CN_205359278_230000_CN_204311935_230000/LConn1 -- T_205359278__/LConn1 -- _CN_205359278_230000_CN_160110669_230000/LConn1
  _CN_205359278_230000_CN_204311935_230000/LConn2 -- T_205359278__/LConn2 -- _CN_205359278_230000_CN_160110669_230000/LConn2
  _CN_205359278_230000_CN_204311935_230000/LConn3 -- T_205359278__/LConn3 -- _CN_205359278_230000_CN_160110669_230000/LConn3 -- bus69/LConn1
  T_204311935__/LConn1 -- _CN_205359278_230000_CN_204311935_230000/RConn1
  T_204311935__/LConn2 -- _CN_205359278_230000_CN_204311935_230000/RConn2
  _CN_205359278_230000_CN_204311935_230000/RConn3 -- T_204311935__/LConn3 -- bus70/LConn1
  _CN_205359278_230000_CN_160110669_230000/RConn1 -- T_160110669__/LConn1 -- _CN_163811126_230000_CN_160110669_230000/LConn1 -- _CN_160110669_230000_CN_160110681_230000/LConn1 -- _CN_151913391_230000_CN_160110669_230000/RConn1
  _CN_205359278_230000_CN_160110669_230000/RConn2 -- T_160110669__/LConn2 -- _CN_163811126_230000_CN_160110669_230000/LConn2 -- _CN_160110669_230000_CN_160110681_230000/LConn2 -- _CN_151913391_230000_CN_160110669_230000/RConn2
  _CN_205359278_230000_CN_160110669_230000/RConn3 -- T_160110669__/LConn3 -- _CN_163811126_230000_CN_160110669_230000/LConn3 -- _CN_160110669_230000_CN_160110681_230000/LConn3 -- bus71/LConn1 -- _CN_151913391_230000_CN_160110669_230000/RConn3
  T_162588721__/LConn1 -- _CN_162588721_230000_CN_133331793_230000/RConn1
  T_162588721__/LConn2 -- _CN_162588721_230000_CN_133331793_230000/RConn2
  _CN_162588721_230000_CN_133331793_230000/RConn3 -- T_162588721__/LConn3 -- bus72/LConn1
  _CN_238298034_230000_CN_330757612_230000/RConn1 -- T_238298034__/LConn1 -- _CN_238298034_230000_CN_382767472_230000/LConn1 -- _CN_238298034_230000_CN_113711692_230000/RConn1
  _CN_238298034_230000_CN_330757612_230000/RConn2 -- T_238298034__/LConn2 -- _CN_238298034_230000_CN_382767472_230000/LConn2 -- _CN_238298034_230000_CN_113711692_230000/RConn2
  _CN_238298034_230000_CN_330757612_230000/RConn3 -- T_238298034__/LConn3 -- _CN_238298034_230000_CN_382767472_230000/LConn3 -- bus73/LConn1 -- _CN_238298034_230000_CN_113711692_230000/RConn3
  T_382767472__/LConn1 -- _CN_238298034_230000_CN_382767472_230000/RConn1
  T_382767472__/LConn2 -- _CN_238298034_230000_CN_382767472_230000/RConn2
  _CN_238298034_230000_CN_382767472_230000/RConn3 -- T_382767472__/LConn3 -- bus74/LConn1
  T_163811126__/LConn1 -- _CN_163811126_230000_CN_160110669_230000/RConn1
  T_163811126__/LConn2 -- _CN_163811126_230000_CN_160110669_230000/RConn2
  _CN_163811126_230000_CN_160110669_230000/RConn3 -- T_163811126__/LConn3 -- bus75/LConn1
  _CN_150974530_230000_CN_150974532_230000/LConn1 -- T_150974530__/RConn1 -- L_150974530/LConn1
  _CN_150974530_230000_CN_150974532_230000/LConn2 -- T_150974530__/RConn2 -- L_150974530/LConn2
  _CN_150974530_230000_CN_150974532_230000/LConn3 -- T_150974530__/RConn3 -- L_150974530/LConn3 -- bus76/LConn1
  _CN_150974530_230000_CN_150974532_230000/RConn1 -- T_150974532__/LConn1 -- _CN_150974532_230000_CN_131661157_230000/LConn1
  _CN_150974530_230000_CN_150974532_230000/RConn2 -- T_150974532__/LConn2 -- _CN_150974532_230000_CN_131661157_230000/LConn2
  _CN_150974530_230000_CN_150974532_230000/RConn3 -- T_150974532__/LConn3 -- _CN_150974532_230000_CN_131661157_230000/LConn3 -- bus77/LConn1
  T_131661157__/LConn1 -- _CN_150974532_230000_CN_131661157_230000/RConn1
  T_131661157__/LConn2 -- _CN_150974532_230000_CN_131661157_230000/RConn2
  _CN_150974532_230000_CN_131661157_230000/RConn3 -- T_131661157__/LConn3 -- bus78/LConn1
  T_133424203__/LConn1 -- _CN_133424203_230000_CN_133424212_230000/RConn1
  T_133424203__/LConn2 -- _CN_133424203_230000_CN_133424212_230000/RConn2
  _CN_133424203_230000_CN_133424212_230000/RConn3 -- T_133424203__/LConn3 -- bus79/LConn1
  _CN_160110669_230000_CN_160110681_230000/RConn1 -- T_160110681__/RConn1 -- L_160110681/LConn1
  _CN_160110669_230000_CN_160110681_230000/RConn2 -- T_160110681__/RConn2 -- L_160110681/LConn2
  _CN_160110669_230000_CN_160110681_230000/RConn3 -- T_160110681__/RConn3 -- L_160110681/LConn3 -- bus80/LConn1
  _CN_133331795_230000_CN_133331793_230000/RConn1 -- T_133331795__/LConn1 -- _CN_133331795_230000_CN_191731888_230000/LConn1
  _CN_133331795_230000_CN_133331793_230000/RConn2 -- T_133331795__/LConn2 -- _CN_133331795_230000_CN_191731888_230000/LConn2
  _CN_133331795_230000_CN_133331793_230000/RConn3 -- T_133331795__/LConn3 -- _CN_133331795_230000_CN_191731888_230000/LConn3 -- bus81/LConn1
  _CN_133331795_230000_CN_191731888_230000/RConn1 -- T_191731888__/RConn1 -- _CN_168164591_230000_CN_191731888_230000/LConn1 -- L_191731888/LConn1
  _CN_133331795_230000_CN_191731888_230000/RConn2 -- T_191731888__/RConn2 -- _CN_168164591_230000_CN_191731888_230000/LConn2 -- L_191731888/LConn2
  _CN_133331795_230000_CN_191731888_230000/RConn3 -- T_191731888__/RConn3 -- _CN_168164591_230000_CN_191731888_230000/LConn3 -- L_191731888/LConn3 -- bus82/LConn1
  _CN_133424212_230000_CN_168164591_230000/RConn1 -- T_168164591__/LConn1 -- _CN_168164591_230000_CN_130593618_230000/RConn1 -- _CN_168164591_230000_CN_191731888_230000/RConn1
  _CN_133424212_230000_CN_168164591_230000/RConn2 -- T_168164591__/LConn2 -- _CN_168164591_230000_CN_130593618_230000/RConn2 -- _CN_168164591_230000_CN_191731888_230000/RConn2
  _CN_133424212_230000_CN_168164591_230000/RConn3 -- T_168164591__/LConn3 -- _CN_168164591_230000_CN_130593618_230000/RConn3 -- _CN_168164591_230000_CN_191731888_230000/RConn3 -- bus83/LConn1
  T_150579316__/LConn1 -- _CN_150358741_230000_CN_150579316_230000/RConn1
  T_150579316__/LConn2 -- _CN_150358741_230000_CN_150579316_230000/RConn2
  _CN_150358741_230000_CN_150579316_230000/RConn3 -- T_150579316__/LConn3 -- bus84/LConn1
  _CN_124803179_230000_CN_154838308_230000/RConn1 -- T_124803179__/LConn1 -- _CN_124803179_230000_CN_130593618_230000/RConn1
  _CN_124803179_230000_CN_154838308_230000/RConn2 -- T_124803179__/LConn2 -- _CN_124803179_230000_CN_130593618_230000/RConn2
  _CN_124803179_230000_CN_154838308_230000/RConn3 -- T_124803179__/LConn3 -- _CN_124803179_230000_CN_130593618_230000/RConn3 -- bus85/LConn1
  _CN_152322304_400000_CN_374038506_400000/LConn1 -- T_152322304__/LConn1 -- _CN_152322304_400000_CN_368996390_400000/LConn1
  _CN_152322304_400000_CN_374038506_400000/LConn2 -- T_152322304__/LConn2 -- _CN_152322304_400000_CN_368996390_400000/LConn2
  _CN_152322304_400000_CN_374038506_400000/LConn3 -- T_152322304__/LConn3 -- _CN_152322304_400000_CN_368996390_400000/LConn3 -- bus86/LConn1
  G_374038506_/RConn1 -- _CN_152322304_400000_CN_374038506_400000/RConn1
  G_374038506_/RConn2 -- _CN_152322304_400000_CN_374038506_400000/RConn2
  _CN_152322304_400000_CN_374038506_400000/RConn3 -- G_374038506_/RConn3 -- bus87/LConn1
  G_368996390_/RConn1 -- _CN_152322304_400000_CN_368996390_400000/RConn1
  G_368996390_/RConn2 -- _CN_152322304_400000_CN_368996390_400000/RConn2
  _CN_152322304_400000_CN_368996390_400000/RConn3 -- G_368996390_/RConn3 -- bus88/LConn1
  T_191731888__/LConn1 -- _CN_191731888_400000_CN_160279731_400000/LConn1
  T_191731888__/LConn2 -- _CN_191731888_400000_CN_160279731_400000/LConn2
  _CN_191731888_400000_CN_160279731_400000/LConn3 -- T_191731888__/LConn3 -- bus89/LConn1
  _CN_191731888_400000_CN_160279731_400000/RConn1 -- T_160279731__/LConn1 -- _CN_150974530_400000_CN_160279731_400000/LConn1
  _CN_191731888_400000_CN_160279731_400000/RConn2 -- T_160279731__/LConn2 -- _CN_150974530_400000_CN_160279731_400000/LConn2
  _CN_191731888_400000_CN_160279731_400000/RConn3 -- T_160279731__/LConn3 -- _CN_150974530_400000_CN_160279731_400000/LConn3 -- bus90/LConn1
  _CN_150974530_400000_CN_160279731_400000/RConn1 -- T_150974530__/LConn1 -- _CN_150974530_400000_CN_130593618_230000/RConn1
  _CN_150974530_400000_CN_160279731_400000/RConn2 -- T_150974530__/LConn2 -- _CN_150974530_400000_CN_130593618_230000/RConn2
  _CN_150974530_400000_CN_160279731_400000/RConn3 -- T_150974530__/LConn3 -- _CN_150974530_400000_CN_130593618_230000/RConn3 -- bus91/LConn1
  _CN_130805767_400000_CN_223083377_400000/LConn1 -- T_130805767__/LConn1 -- _CN_130805767_400000_CN_307736698_400000/LConn1
  _CN_130805767_400000_CN_223083377_400000/LConn2 -- T_130805767__/LConn2 -- _CN_130805767_400000_CN_307736698_400000/LConn2
  _CN_130805767_400000_CN_223083377_400000/LConn3 -- T_130805767__/LConn3 -- _CN_130805767_400000_CN_307736698_400000/LConn3 -- bus92/LConn1
  T_223083377__/LConn1 -- _CN_130805767_400000_CN_223083377_400000/RConn1
  T_223083377__/LConn2 -- _CN_130805767_400000_CN_223083377_400000/RConn2
  _CN_130805767_400000_CN_223083377_400000/RConn3 -- T_223083377__/LConn3 -- bus93/LConn1
  _CN_130805767_400000_CN_307736698_400000/RConn1 -- T_307736698__/LConn1 -- _CN_150638744_400000_CN_307736698_400000/LConn1
  _CN_130805767_400000_CN_307736698_400000/RConn2 -- T_307736698__/LConn2 -- _CN_150638744_400000_CN_307736698_400000/LConn2
  _CN_130805767_400000_CN_307736698_400000/RConn3 -- T_307736698__/LConn3 -- _CN_150638744_400000_CN_307736698_400000/LConn3 -- bus94/LConn1
  T_117335600_400000;230000_/LConn1 -- _CN_117335600_400000_CN_160110681_400000/LConn1
  T_117335600_400000;230000_/LConn2 -- _CN_117335600_400000_CN_160110681_400000/LConn2
  _CN_117335600_400000_CN_160110681_400000/LConn3 -- T_117335600_400000;230000_/LConn3 -- bus95/LConn1
  _CN_117335600_400000_CN_160110681_400000/RConn1 -- T_160110681__/LConn1 -- _CN_150638744_400000_CN_160110681_400000/LConn1 -- _CN_160110681_400000_CN_163808669_400000/LConn1
  _CN_117335600_400000_CN_160110681_400000/RConn2 -- T_160110681__/LConn2 -- _CN_150638744_400000_CN_160110681_400000/LConn2 -- _CN_160110681_400000_CN_163808669_400000/LConn2
  _CN_117335600_400000_CN_160110681_400000/RConn3 -- T_160110681__/LConn3 -- _CN_150638744_400000_CN_160110681_400000/LConn3 -- _CN_160110681_400000_CN_163808669_400000/LConn3 -- bus96/LConn1
  _CN_150638744_400000_CN_130593618_230000/RConn1 -- T_150638744__/LConn1 -- _CN_150638744_400000_CN_307736698_400000/RConn1 -- _CN_150638744_400000_CN_160110681_400000/RConn1
  _CN_150638744_400000_CN_130593618_230000/RConn2 -- T_150638744__/LConn2 -- _CN_150638744_400000_CN_307736698_400000/RConn2 -- _CN_150638744_400000_CN_160110681_400000/RConn2
  _CN_150638744_400000_CN_130593618_230000/RConn3 -- T_150638744__/LConn3 -- _CN_150638744_400000_CN_307736698_400000/RConn3 -- bus97/LConn1 -- _CN_150638744_400000_CN_160110681_400000/RConn3
  T_163808669__/LConn1 -- _CN_160110681_400000_CN_163808669_400000/RConn1
  T_163808669__/LConn2 -- _CN_160110681_400000_CN_163808669_400000/RConn2
  _CN_160110681_400000_CN_163808669_400000/RConn3 -- T_163808669__/LConn3 -- bus98/LConn1
  T_172436615__/RConn1 -- L_172436615/LConn1
  T_172436615__/RConn2 -- L_172436615/LConn2
  L_172436615/LConn3 -- T_172436615__/RConn3 -- bus99/LConn1
  T_150358740__/RConn1 -- L_150358740/LConn1
  T_150358740__/RConn2 -- L_150358740/LConn2
  L_150358740/LConn3 -- T_150358740__/RConn3 -- bus100/LConn1
  T_152303368__/RConn1 -- L_152303368/LConn1
  T_152303368__/RConn2 -- L_152303368/LConn2
  L_152303368/LConn3 -- T_152303368__/RConn3 -- bus101/LConn1
  T_152322299__/RConn1 -- L_152322299/LConn1
  T_152322299__/RConn2 -- L_152322299/LConn2
  L_152322299/LConn3 -- T_152322299__/RConn3 -- bus102/LConn1
  T_223610661__/RConn1 -- L_223610661/LConn1
  T_223610661__/RConn2 -- L_223610661/LConn2
  L_223610661/LConn3 -- T_223610661__/RConn3 -- bus103/LConn1
  T_130790482__/RConn1 -- L_130790482/LConn1
  T_130790482__/RConn2 -- L_130790482/LConn2
  L_130790482/LConn3 -- T_130790482__/RConn3 -- bus104/LConn1
  T_382319714__/RConn1 -- L_382319714/LConn1
  T_382319714__/RConn2 -- L_382319714/LConn2
  L_382319714/LConn3 -- T_382319714__/RConn3 -- bus105/LConn1
  T_154474061__/RConn1 -- L_154474061/LConn1
  T_154474061__/RConn2 -- L_154474061/LConn2
  L_154474061/LConn3 -- T_154474061__/RConn3 -- bus106/LConn1
  T_153750231__/RConn1 -- L_153750231/LConn1
  T_153750231__/RConn2 -- L_153750231/LConn2
  L_153750231/LConn3 -- T_153750231__/RConn3 -- bus107/LConn1
  T_204550424__/RConn1 -- L_204550424/LConn1
  T_204550424__/RConn2 -- L_204550424/LConn2
  L_204550424/LConn3 -- T_204550424__/RConn3 -- bus108/LConn1
  T_180330721__/RConn1 -- L_180330721/LConn1
  T_180330721__/RConn2 -- L_180330721/LConn2
  L_180330721/LConn3 -- T_180330721__/RConn3 -- bus109/LConn1
  T_368593331__/RConn1 -- L_368593331/LConn1
  T_368593331__/RConn2 -- L_368593331/LConn2
  L_368593331/LConn3 -- T_368593331__/RConn3 -- bus110/LConn1
  T_171978321__/RConn1 -- L_171978321/LConn1
  T_171978321__/RConn2 -- L_171978321/LConn2
  L_171978321/LConn3 -- T_171978321__/RConn3 -- bus111/LConn1
  T_167991716_66000_/RConn1 -- L_167991716/LConn1
  T_167991716_66000_/RConn2 -- L_167991716/LConn2
  L_167991716/LConn3 -- T_167991716_66000_/RConn3 -- bus112/LConn1
  T_157393020__/RConn1 -- L_157393020/LConn1
  T_157393020__/RConn2 -- L_157393020/LConn2
  L_157393020/LConn3 -- T_157393020__/RConn3 -- bus113/LConn1
  T_223610662__/RConn1 -- L_223610662/LConn1
  T_223610662__/RConn2 -- L_223610662/LConn2
  L_223610662/LConn3 -- T_223610662__/RConn3 -- bus114/LConn1
  T_382300120__/RConn1 -- L_382300120/LConn1
  T_382300120__/RConn2 -- L_382300120/LConn2
  L_382300120/LConn3 -- T_382300120__/RConn3 -- bus115/LConn1
  T_382331561__/RConn1 -- L_382331561/LConn1
  T_382331561__/RConn2 -- L_382331561/LConn2
  L_382331561/LConn3 -- T_382331561__/RConn3 -- bus116/LConn1
  T_382898922__/RConn1 -- L_382898922/LConn1
  T_382898922__/RConn2 -- L_382898922/LConn2
  L_382898922/LConn3 -- T_382898922__/RConn3 -- bus117/LConn1
  T_382484415__/RConn1 -- L_382484415/LConn1
  T_382484415__/RConn2 -- L_382484415/LConn2
  L_382484415/LConn3 -- T_382484415__/RConn3 -- bus118/LConn1
  T_155496431__/RConn1 -- L_155496431/LConn1
  T_155496431__/RConn2 -- L_155496431/LConn2
  L_155496431/LConn3 -- T_155496431__/RConn3 -- bus119/LConn1
  T_171978319__/RConn1 -- L_171978319/LConn1
  T_171978319__/RConn2 -- L_171978319/LConn2
  L_171978319/LConn3 -- T_171978319__/RConn3 -- bus120/LConn1
  T_160840191__/RConn1 -- L_160840191/LConn1
  T_160840191__/RConn2 -- L_160840191/LConn2
  L_160840191/LConn3 -- T_160840191__/RConn3 -- bus121/LConn1
  T_163711729__/RConn1 -- L_163711729/LConn1
  T_163711729__/RConn2 -- L_163711729/LConn2
  L_163711729/LConn3 -- T_163711729__/RConn3 -- bus122/LConn1
  T_110461432__محطة_الكهرباء/RConn1 -- L_110461432/LConn1
  T_110461432__محطة_الكهرباء/RConn2 -- L_110461432/LConn2
  L_110461432/LConn3 -- T_110461432__محطة_الكهرباء/RConn3 -- bus123/LConn1
  T_161969636__/RConn1 -- L_161969636/LConn1
  T_161969636__/RConn2 -- L_161969636/LConn2
  L_161969636/LConn3 -- T_161969636__/RConn3 -- bus124/LConn1
  T_164725547__/RConn1 -- L_164725547/LConn1
  T_164725547__/RConn2 -- L_164725547/LConn2
  L_164725547/LConn3 -- T_164725547__/RConn3 -- bus125/LConn1
  T_195237417__/RConn1 -- L_195237417/LConn1
  T_195237417__/RConn2 -- L_195237417/LConn2
  L_195237417/LConn3 -- T_195237417__/RConn3 -- bus126/LConn1
  T_152303369__/RConn1 -- L_152303369/LConn1
  T_152303369__/RConn2 -- L_152303369/LConn2
  L_152303369/LConn3 -- T_152303369__/RConn3 -- bus127/LConn1
  T_254292628__/RConn1 -- L_254292628/LConn1
  T_254292628__/RConn2 -- L_254292628/LConn2
  L_254292628/LConn3 -- T_254292628__/RConn3 -- bus128/LConn1
  T_133424212__/RConn1 -- L_133424212/LConn1
  T_133424212__/RConn2 -- L_133424212/LConn2
  L_133424212/LConn3 -- T_133424212__/RConn3 -- bus129/LConn1
  T_254292629__/RConn1 -- L_254292629/LConn1
  T_254292629__/RConn2 -- L_254292629/LConn2
  L_254292629/LConn3 -- T_254292629__/RConn3 -- bus130/LConn1
  T_151913391__/RConn1 -- L_151913391/LConn1
  T_151913391__/RConn2 -- L_151913391/LConn2
  L_151913391/LConn3 -- T_151913391__/RConn3 -- bus131/LConn1
  T_150358741__/RConn1 -- L_150358741/LConn1
  T_150358741__/RConn2 -- L_150358741/LConn2
  L_150358741/LConn3 -- T_150358741__/RConn3 -- bus132/LConn1
  T_330757612__/RConn1 -- L_330757612/LConn1
  T_330757612__/RConn2 -- L_330757612/LConn2
  L_330757612/LConn3 -- T_330757612__/RConn3 -- bus133/LConn1
  T_180326309__Electrical_substation/RConn1 -- L_180326309/LConn1
  T_180326309__Electrical_substation/RConn2 -- L_180326309/LConn2
  L_180326309/LConn3 -- T_180326309__Electrical_substation/RConn3 -- bus134/LConn1
  T_113711692__/RConn1 -- L_113711692/LConn1
  T_113711692__/RConn2 -- L_113711692/LConn2
  L_113711692/LConn3 -- T_113711692__/RConn3 -- bus135/LConn1
  T_123913890__/RConn1 -- L_123913890/LConn1
  T_123913890__/RConn2 -- L_123913890/LConn2
  L_123913890/LConn3 -- T_123913890__/RConn3 -- bus136/LConn1
  T_130592294__/RConn1 -- L_130592294/LConn1
  T_130592294__/RConn2 -- L_130592294/LConn2
  L_130592294/LConn3 -- T_130592294__/RConn3 -- bus137/LConn1
  T_164701658__/RConn1 -- L_164701658/LConn1
  T_164701658__/RConn2 -- L_164701658/LConn2
  L_164701658/LConn3 -- T_164701658__/RConn3 -- bus138/LConn1
  T_133432875__/RConn1 -- L_133432875/LConn1
  T_133432875__/RConn2 -- L_133432875/LConn2
  L_133432875/LConn3 -- T_133432875__/RConn3 -- bus139/LConn1
  T_205359278__/RConn1 -- L_205359278/LConn1
  T_205359278__/RConn2 -- L_205359278/LConn2
  L_205359278/LConn3 -- T_205359278__/RConn3 -- bus140/LConn1
  T_204311935__/RConn1 -- L_204311935/LConn1
  T_204311935__/RConn2 -- L_204311935/LConn2
  L_204311935/LConn3 -- T_204311935__/RConn3 -- bus141/LConn1
  T_160110669__/RConn1 -- L_160110669/LConn1
  T_160110669__/RConn2 -- L_160110669/LConn2
  L_160110669/LConn3 -- T_160110669__/RConn3 -- bus142/LConn1
  T_162588721__/RConn1 -- L_162588721/LConn1
  T_162588721__/RConn2 -- L_162588721/LConn2
  L_162588721/LConn3 -- T_162588721__/RConn3 -- bus143/LConn1
  T_382767472__/RConn1 -- L_382767472/LConn1
  T_382767472__/RConn2 -- L_382767472/LConn2
  L_382767472/LConn3 -- T_382767472__/RConn3 -- bus144/LConn1
  T_163811126__/RConn1 -- L_163811126/LConn1
  T_163811126__/RConn2 -- L_163811126/LConn2
  L_163811126/LConn3 -- T_163811126__/RConn3 -- bus145/LConn1
  T_131661157__/RConn1 -- L_131661157/LConn1
  T_131661157__/RConn2 -- L_131661157/LConn2
  L_131661157/LConn3 -- T_131661157__/RConn3 -- bus146/LConn1
  T_133424203__/RConn1 -- L_133424203/LConn1
  T_133424203__/RConn2 -- L_133424203/LConn2
  L_133424203/LConn3 -- T_133424203__/RConn3 -- bus147/LConn1
  T_168164591__/RConn1 -- L_168164591/LConn1
  T_168164591__/RConn2 -- L_168164591/LConn2
  L_168164591/LConn3 -- T_168164591__/RConn3 -- bus148/LConn1
  T_150579316__/RConn1 -- L_150579316/LConn1
  T_150579316__/RConn2 -- L_150579316/LConn2
  L_150579316/LConn3 -- T_150579316__/RConn3 -- bus149/LConn1
  T_124803179__/RConn1 -- L_124803179/LConn1
  T_124803179__/RConn2 -- L_124803179/LConn2
  L_124803179/LConn3 -- T_124803179__/RConn3 -- bus150/LConn1
  T_223083377__/RConn1 -- L_223083377/LConn1
  T_223083377__/RConn2 -- L_223083377/LConn2
  L_223083377/LConn3 -- T_223083377__/RConn3 -- bus151/LConn1
  T_307736698__/RConn1 -- L_307736698/LConn1
  T_307736698__/RConn2 -- L_307736698/LConn2
  L_307736698/LConn3 -- T_307736698__/RConn3 -- bus152/LConn1
  T_163808669__/RConn1 -- L_163808669/LConn1
  T_163808669__/RConn2 -- L_163808669/LConn2
  L_163808669/LConn3 -- T_163808669__/RConn3 -- bus153/LConn1
